simulink model "first"  (R2020a)
settings: Solver=VariableStepAuto  StartTime=0.0  StopTime=10.0  RelTol=1e-3
settings Model: Creator=pc  LastModifiedBy=pc

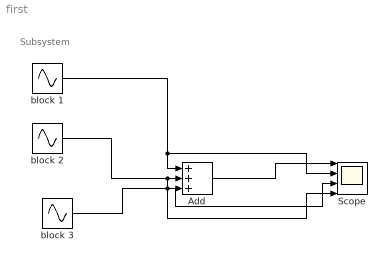
== system first ==
  note: Subsystem
  Add : Sum  Inputs=+++
  Scope : Scope  NumInputPorts=4
  block 1 : Sin  Amplitude=4  SampleTime=0
  block 2 : Sin  Amplitude=3  SampleTime=0
  block 3 : Sin  SampleTime=0
  wires:
  block 2/1 -> Scope/4, Add/2
  Add/1 -> Scope/1
  block 1/1 -> Add/1, Scope/2
  block 3/1 -> Scope/3, Add/3
